simulink model "test_ac_controller"  (R2023b)
settings: Solver=FixedStepAuto  StartTime=0.0  StopTime=10.0  RelTol=1e-3
libraries: ac_controller x1
settings Model: Creator=kilia  LastModifiedBy=kilia
settings HardwareCC: TargetBitPerPointer=64  TargetBitPerSizeT=64  TargetBitPerPtrDiffT=64  TargetLongLongMode=on  TargetIntDivRoundTo=Zero  TargetEndianess=LittleEndian  TargetWordSize=64  TargetHWDeviceType=MATLAB Host  ProdEqTarget=off
settings RTWCC: Description=S-Function Target  SystemTargetFile=rtwsfcn.tlc  TemplateMakefile=rtwsfcn_default_tmf
settings STFCustomTargetCC: ModelReferenceCompliant=off  CompOptLevelCompliant=on  MATLABClassNameForMDSCustomization=Simulink.SoftwareTarget.TargetSpecificTriggerConfigurationBase  GRTInterface=on  SystemTargetFile=rtwsfcn.tlc

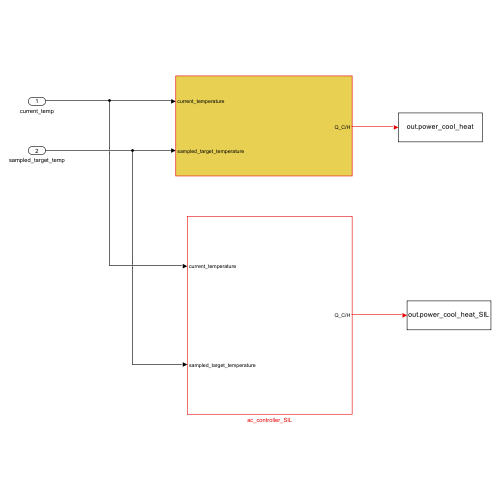
[thumbnail: Simulink's stored preview of the top-level diagram]
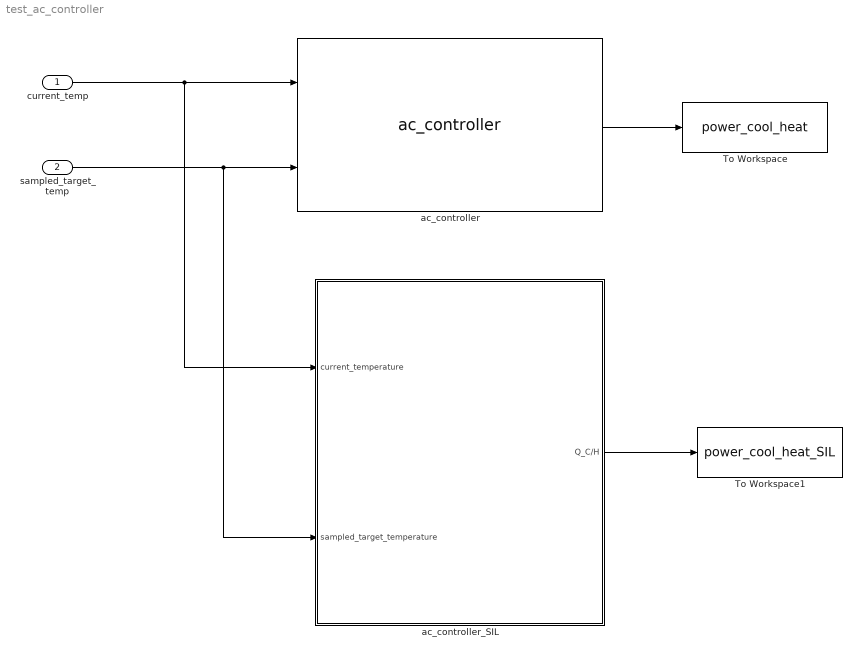
== system test_ac_controller ==
  current_temp : Inport  OutDataTypeStr=int16  SampleTime=0.1  Interpolate=off
  sampled_target_temp : Inport  Port=2  OutDataTypeStr=int16  SampleTime=0.1  Interpolate=off
  To Workspace : ToWorkspace  VariableName=power_cool_heat  SaveFormat=Timeseries  SampleTime=-1
  To Workspace1 : ToWorkspace  VariableName=power_cool_heat_SIL  SaveFormat=Timeseries  SampleTime=-1
  ac_controller : ac_controller/ac_controller  SystemSampleTime=-1  VariantActivationTime=update diagram  AllowFlexibleInterface=on  Latency=0  AutoFrameSizeCalculation=off
  ac_controller_SIL : Subsystem
      mask help: Simulink:masks:GenSFuncDesc_MD
      mask Help: eval('feval(''rtwprivate'',''rtwhelpview'',''rtw_sfcn_block'')');
  wires:
  sampled_target_temp/1 -> ac_controller_SIL/2(sampled_target_temperature), ac_controller/2
  ac_controller/1 -> To Workspace/1
  current_temp/1 -> ac_controller_SIL/1(current_temperature), ac_controller/1
  ac_controller_SIL/1(Q_C/H) -> To Workspace1/1

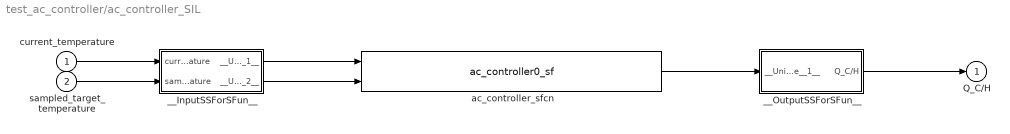
== system test_ac_controller/ac_controller_SIL ==
  current_temperature : Inport
  sampled_target_temperature : Inport  Port=2
  __InputSSForSFun__ : Subsystem
  __OutputSSForSFun__ : Subsystem
  ac_controller_sfcn : S-Function  FunctionName=ac_controller0_sf  SFunctionModules=""  SFunctionDeploymentMode=off  EnableBusSupport=off  SFcnStateName=DWORK0  mask{rtw_sf_name=ac_controller0_sf, showVar=off}
      mask prompts: rtw_sf_name "Simulink:masks:GenSFuncName_MP"; showVar "Simulink:masks:GenSFuncShowModuleList_MP"
      mask help: Simulink:masks:GenSFuncDesc_MD
      mask init:
      | displist = '';
      | if ~strcmp(get_param(gcb, 'FunctionName'), rtw_sf_name);
      |   set_param(gcb, 'FunctionName', rtw_sf_name);
      | end
      | % Check if we are generating code
      | rtw_mode = false;
      | if strcmpi(get_param(bdroot(gcb),'SimulationStatus'),'Initializing')
      | 	rtw_mode = strcmpi(get_param(bdroot(gcb),'BuildingRTWCode'),'on') && ...
      | 		~strcmpi(get_param(bdroot(gcb),'TargetStyle'),'SimulationTarget');
      | end
      | if showVar || rtw_mode
      | 	if exist('rtwsfunc') == 2 | exist('rtwsfunc') == 6
      | 		tmplist = rtwsfunc(rtw_sf_name,gcb);
      | 		tmplist = DAStudio.message('Simulink:masks:GenSFuncListOfModules_IC', tmplist);
      | 	elseif showVar
      | 		tmplist1 = DAStudio.message('Simulink:masks:GenSFuncListOfModules_IC', '');
      |         tmplist2 = DAStudio.message('Simulink:masks:GenSFuncNotLicensed_IC');
      |         tmplist = [tmplist1 tmplist2];
      |  	end
      | end
      | if showVar
      |   displist = tmplist;
      | end
      settings: SFcnIsStateOwnerBlock=on
      settings: CopyFcn=|
      | if ~strcmp(get_param(gcb,'Linkstatus'),'none') && ...
      | ~strcmp(get_param(gcb,'Linkstatus'),'implicit')
      |   set_param(gcb,'LinkStatus','none');
      | end
      mask Help: eval('feval(''rtwprivate'',''rtwhelpview'',''rtw_sfcn_block'')');
      mask Display:
      | port_label('input',1,'current_temperature');
      | port_label('input',2,'sampled_target_temperature');
      | port_label('output',1,'Q_C/H');
  Q_C/H : Outport  LockScale=on
  wires:
  __OutputSSForSFun__/1(Q_C/H) -> Q_C/H/1
  ac_controller_sfcn/1 -> __OutputSSForSFun__/1(__UniqueInportName__1__)
  __InputSSForSFun__/2(__UniqueOutportName__2__) -> ac_controller_sfcn/2
  __InputSSForSFun__/1(__UniqueOutportName__1__) -> ac_controller_sfcn/1
  sampled_target_temperature/1 -> __InputSSForSFun__/2(sampled_target_temperature)
  current_temperature/1 -> __InputSSForSFun__/1(current_temperature)

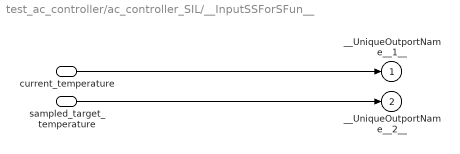
== system test_ac_controller/ac_controller_SIL/__InputSSForSFun__ ==
  current_temperature : Inport
  sampled_target_temperature : Inport  Port=2
  __UniqueOutportName__1__ : Outport
  __UniqueOutportName__2__ : Outport  Port=2
  wires:
  sampled_target_temperature/1 -> __UniqueOutportName__2__/1
  current_temperature/1 -> __UniqueOutportName__1__/1

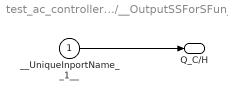
== system test_ac_controller/ac_controller_SIL/__OutputSSForSFun__ ==
  __UniqueInportName__1__ : Inport
  Q_C/H : Outport  LockScale=on
  wires:
  __UniqueInportName__1__/1 -> Q_C/H/1
